simulink model "Practica1"  (R2025b)
settings: Solver=VariableStepAuto  StartTime=0.0  StopTime=30.0  RelTol=1e-3

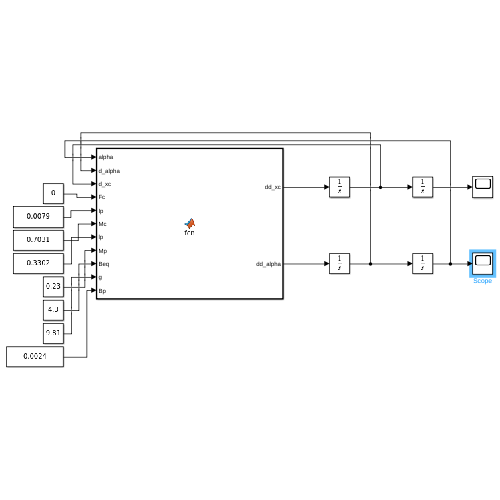
[thumbnail: Simulink's stored preview of the top-level diagram]
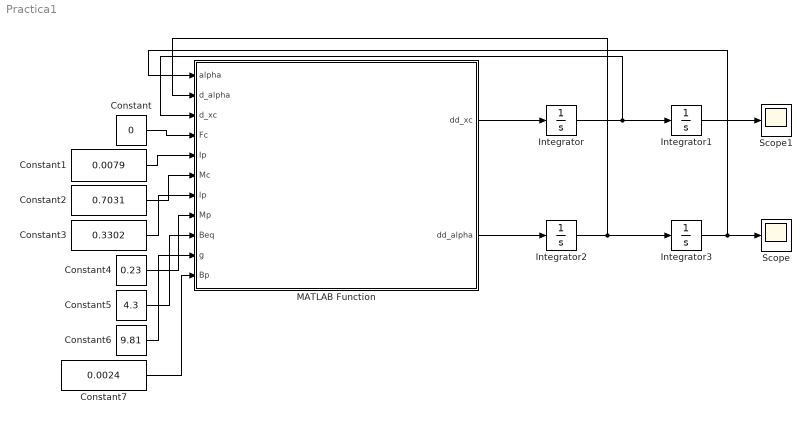
== system Practica1 ==
  Constant : Constant  Value=0
  Constant1 : Constant  Value=0.0079
  Constant2 : Constant  Value=0.7031
  Constant3 : Constant  Value=0.3302
  Constant4 : Constant  Value=0.23
  Constant5 : Constant  Value=4.3
  Constant6 : Constant  Value=9.81
  Constant7 : Constant  Value=0.0024
  Integrator : Integrator
  Integrator1 : Integrator
  Integrator2 : Integrator
  Integrator3 : Integrator  InitialCondition=1 * pi / 180
  MATLAB Function : MATLAB Function  TreatAsAtomicUnit=on
  Scope : Scope
      settings: ActiveDisplayYMinimum=-1.7022068027651018  ActiveDisplayYMaximum=6.0643303819860312
  Scope1 : Scope
      settings: ActiveDisplayYMinimum=-0.12462441142685114  ActiveDisplayYMaximum=0.62421229047384619
  wires:
  MATLAB Function/2(dd_alpha) -> Integrator2/1
  MATLAB Function/1(dd_xc) -> Integrator/1
  Integrator2/1 -> MATLAB Function/2(d_alpha), Integrator3/1
  Integrator/1 -> MATLAB Function/3(d_xc), Integrator1/1
  Integrator3/1 -> Scope/1, MATLAB Function/1(alpha)
  Constant/1 -> MATLAB Function/4(Fc)
  Constant1/1 -> MATLAB Function/5(Ip)
  Constant2/1 -> MATLAB Function/6(Mc)
  Constant3/1 -> MATLAB Function/7(lp)
  Constant4/1 -> MATLAB Function/8(Mp)
  Constant5/1 -> MATLAB Function/9(Beq)
  Constant6/1 -> MATLAB Function/10(g)
  Constant7/1 -> MATLAB Function/11(Bp)
  Integrator1/1 -> Scope1/1

== matlab function Practica1/MATLAB Function ==
  data: alpha input; dd_xc output; d_alpha input; d_xc input; Fc input; Ip input; Mc input; lp input; Mp input; Beq input; g input; Bp input; dd_alpha output
function [dd_xc, dd_alpha] = fcn(alpha, d_alpha, d_xc, Fc, Ip, Mc, lp, Mp, Beq, g, Bp)

den = (Mc + Mp)*Ip + Mc*Mp*lp^2 + Mp^2*lp^2*sin(alpha)^2;

num1 = (Ip + Mp*lp^2)*Fc ...
     + Mp^2*lp^2*g*cos(alpha)*sin(alpha) ...
     - (Ip + Mp*lp^2)*Beq*d_xc ...
     - (Ip*Mp*lp + Mp^2*lp^3)*d_alpha^2*sin(alpha) ...
     - Mp*lp*d_alpha*cos(alpha)*Bp;

dd_xc = num1 / den;

num2 = (Mc + Mp)*Mp*g*lp*sin(alpha) ...
     - (Mc + Mp)*Bp*d_alpha ...
     + Fc*Mp*lp*cos(alpha) ...
     - Mp^2*lp^2*d_alpha^2*sin(alpha)*cos(alpha) ...
     - Beq*Mp*lp*d_xc*cos(alpha);

dd_alpha = num2 / den;

end
